simulink model "fb_lin_test_612_sec"  (R2020b)
settings: Solver=VariableStepAuto  StartTime=0.0  StopTime=10.0  RelTol=1e-3
settings Model: Creator=ASUS  LastModifiedBy=ASUS

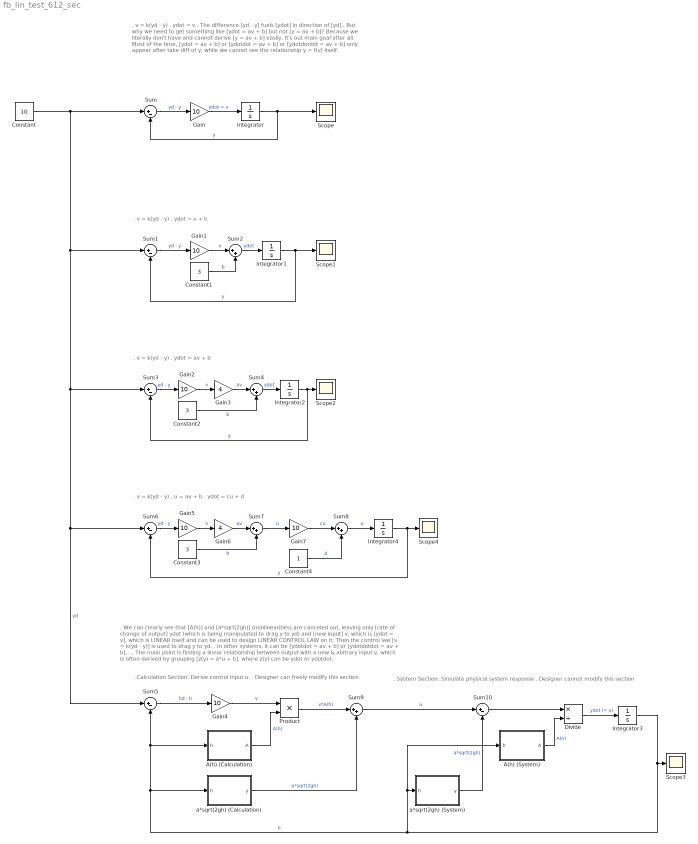
== system fb_lin_test_612_sec ==
  note: . We can clearly see that [A(h)] and [a*sqrt(2gh)] (nonlinearities) are canceled out, leaving only [rate of change of output] ydot (which is being manipulated to drag y to yd) and
      | [new input] v, which is [ydot = v], which is LINEAR itself and can be used to design LINEAR CONTROL LAW on it. Then the control law [v = k(yd - y)] is used to drag y to yd.
      |
      | . In other systems, it can be [ydotdot = av + b] or  [ydotdotdot = av + b], ... The main point is finding a linear relationship between output with a new & abitrary input v, which is often
      | derived by grouping [z(y) = a*u + b], where z(y) can be ydot or ydotdot.
  note: . System Section: Simulate physical system response
      | . Designer cannot modify this section
  note: . Calculation Section: Derive control input u.
      | . Designer can freely modify this section
  note: . v = k(yd - y)
      | . ydot = v + b
  note: . v = k(yd - y)
      | . ydot = v
      | . The difference [yd - y] fuels [ydot] in direction of [yd]
      | . But why we need to get something like [ydot = av + b] but
      | not [y = av + b]? Because we literally don't have and cannot
      | derive  [y = av + b] easliy. It's out main goal after all. Most of the
      |  time, [ydot = av + b] or [ydotdot = av + b] or
      | [ydotdotdot = av + b] only appear after take diff of y, while we
      | cannot see the relationship y = f(v) itself.
  note: . v = k(yd - y)
      | . ydot = av + b
  note: . v = k(yd - y)
      | . u = av + b
      | . ydot = cu + d
  A(h) (Calculation) : MATLAB Function  TreatAsAtomicUnit=on
  A(h) (System) : MATLAB Function  TreatAsAtomicUnit=on
  Constant : Constant  Value=10
  Constant1 : Constant  Value=3
  Constant2 : Constant  Value=3
  Constant3 : Constant  Value=3
  Constant4 : Constant
  Divide : Product  Inputs=*/
  Gain{,1..2,4..5,7} (6 alike) : Gain  Gain=10
  Gain3 : Gain  Gain=4
  Gain6 : Gain  Gain=4
  Integrator{,1..4} (5 alike) : Integrator
  Product : Product
  Scope{,1..4} (5 alike) : Scope
  Sum{,1,3,5..6,10} (6 alike) : Sum  Inputs=|+-
  Sum{2,4,7..9} (5 alike) : Sum  Inputs=|++
  a*sqrt(2gh) (Calculation) : MATLAB Function  TreatAsAtomicUnit=on
  a*sqrt(2gh) (System) : MATLAB Function  TreatAsAtomicUnit=on
  wires:
  Constant/1 -> Sum5/1, Sum6/1, Sum3/1, Sum1/1, Sum/1  "yd"
  Integrator/1 -> Scope/1, Sum/2  "y"
  Sum/1 -> Gain/1  "yd - y"
  Gain/1 -> Integrator/1  "ydot = v"
  Sum1/1 -> Gain1/1  "yd - y"
  Gain1/1 -> Sum2/1  "v"
  Constant1/1 -> Sum2/2  "b"
  Sum2/1 -> Integrator1/1  "ydot"
  Integrator1/1 -> Scope1/1, Sum1/2  "y"
  Integrator2/1 -> Scope2/1, Sum3/2  "y"
  Gain2/1 -> Gain3/1  "v"
  Constant2/1 -> Sum4/2  "b"
  Sum3/1 -> Gain2/1  "yd - y"
  Sum4/1 -> Integrator2/1  "ydot"
  Gain3/1 -> Sum4/1  "av"
  Integrator3/1 -> Scope3/1, A(h) (System)/1(h), a*sqrt(2gh) (System)/1(h), Sum5/2, A(h) (Calculation)/1(h), a*sqrt(2gh) (Calculation)/1(h)  "h"
  Sum5/1 -> Gain4/1  "hd - h"
  Gain4/1 -> Product/1  "v"
  Gain5/1 -> Gain6/1  "v"
  Integrator4/1 -> Scope4/1, Sum6/2  "y"
  Gain6/1 -> Sum7/1  "av"
  Constant3/1 -> Sum7/2  "b"
  Sum6/1 -> Gain5/1  "yd - y"
  Sum7/1 -> Gain7/1  "u"
  Gain7/1 -> Sum8/1  "cu"
  Constant4/1 -> Sum8/2  "d"
  Sum8/1 -> Integrator4/1  "u"
  Product/1 -> Sum9/1  "v*A(h)"
  A(h) (Calculation)/1(A) -> Product/2  "A(h)"
  a*sqrt(2gh) (Calculation)/1(y) -> Sum9/2  "a*sqrt(2gh)"
  Sum9/1 -> Sum10/1  "u"
  Sum10/1 -> Divide/1
  a*sqrt(2gh) (System)/1(y) -> Sum10/2  "a*sqrt(2gh)"
  A(h) (System)/1(A) -> Divide/2  "A(h)"
  Divide/1 -> Integrator3/1  "ydot (= v)"

== matlab function fb_lin_test_612_sec/A(h) (Calculation) ==
  data: h input; A output
function A = fcn(h)

A = 0*h + 3;

== matlab function fb_lin_test_612_sec/A(h) (System) ==
  data: h input; A output
function A = fcn(h)

A = 0*h + 3;

== matlab function fb_lin_test_612_sec/a*sqrt(2gh) (System) ==
  data: h input; y output
function y = fcn(h)

a = 1;
g = 9.81;

y = a*sqrt(2*g*h);

== matlab function fb_lin_test_612_sec/a*sqrt(2gh) (Calculation) ==
  data: h input; y output
function y = fcn(h)

a = 1;
g = 9.81;

y = a*sqrt(2*g*h);
